simulink model "lab5PreLab"  (R2020a)
settings: Solver=ode4  StartTime=0.0  StopTime=10.0  FixedStep=0.001  RelTol=1e-3
undefined symbols (not defined in the file): AA, BB, CC, DD, ramp_amp, ramp_start, ramp_tot
libraries: lab5Library x1
settings Model: Creator=ggparker-adm  LastModifiedBy=Ross
settings DataIOCC: ReturnWorkspaceOutputs=off
settings DebuggingCC: ArithmeticOperatorsInVariantConditions=warning
settings SFSimCC: SimUseLocalCustomCode=off  CustomCodeUndefinedFunction=UseInterfaceOnly
settings RTWCC: RTWUseLocalCustomCode=off
settings CodeAppCC: StateflowObjectComments=on

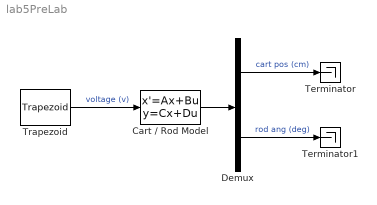
== system lab5PreLab ==
  Cart / Rod Model : StateSpace  A=AA  B=BB  C=CC  D=DD  InitialCondition=[0;0;0;0]
  Demux : Demux  Outputs=2
  Terminator : Terminator
  Terminator1 : Terminator
  Trapezoid : lab5Library/Trapezoid  A=ramp_amp  Ts=ramp_start  Tr=ramp_time  T=ramp_tot
  wires:
  Cart / Rod Model/1 -> Demux/1
  Demux/1 -> Terminator/1  "cart pos (cm)"
  Demux/2 -> Terminator1/1  "rod ang (deg)"
  Trapezoid/1 -> Cart / Rod Model/1  "voltage (v)"
